simulink model "TST_Rail_CtlLoopLimMeUn"  (R2016b)
settings: Solver=FixedStepDiscrete  StartTime=0.0  StopTime=simTime  FixedStep=sampleTime  RelTol=1e-3
values from neighbouring files (symbols this model uses):
  testCase = 1    [initTST_Rail_CtlLoopLimMeUn_001.m]
libraries: simulink x3, UnitTest_Lib x1
settings Model: Creator=zhengjinyan  LastModifiedBy=zhengjinyan
settings DebuggingCC: SignalRangeChecking=error

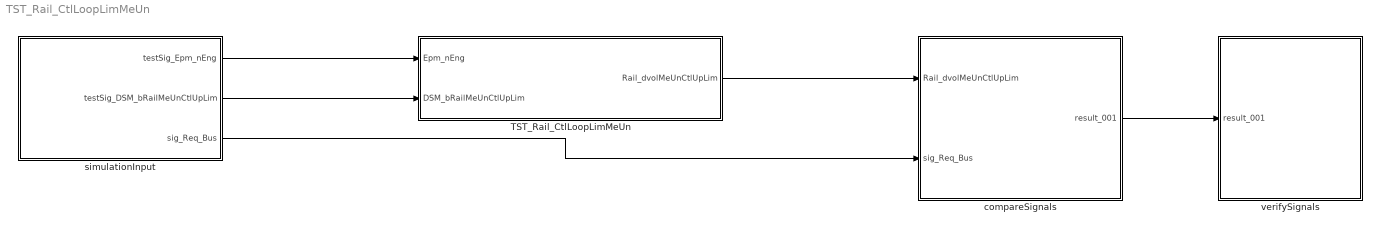
== system TST_Rail_CtlLoopLimMeUn ==
  TST_Rail_CtlLoopLimMeUn : Subsystem
  compareSignals : Subsystem
  simulationInput : Subsystem
  verifySignals : Subsystem
  wires:
  simulationInput/1(testSig_Epm_nEng) -> TST_Rail_CtlLoopLimMeUn/1(Epm_nEng)
  simulationInput/2(testSig_DSM_bRailMeUnCtlUpLim) -> TST_Rail_CtlLoopLimMeUn/2(DSM_bRailMeUnCtlUpLim)
  TST_Rail_CtlLoopLimMeUn/1(Rail_dvolMeUnCtlUpLim) -> compareSignals/1(Rail_dvolMeUnCtlUpLim)
  simulationInput/3(sig_Req_Bus) -> compareSignals/2(sig_Req_Bus)
  compareSignals/1(result_001) -> verifySignals/1(result_001)

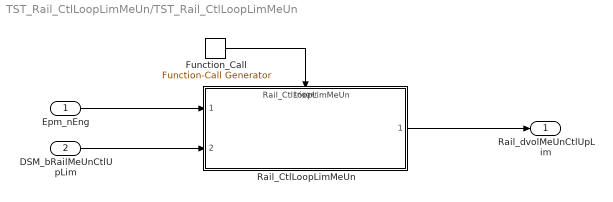
== system TST_Rail_CtlLoopLimMeUn/TST_Rail_CtlLoopLimMeUn ==
  Epm_nEng : Inport
  DSM_bRailMeUnCtlUpLim : Inport  Port=2
  Function_Call : simulink/Ports & Subsystems/Function-Call Generator  sample_time=sampleTime  numberOfIterations=1
  Rail_CtlLoopLimMeUn : ModelReference  ModelNameDialog=Rail_CtlLoopLimMeUn  SimulationMode=Normal  ModelReferenceVersion=1.5  TriggerPortName=function  TriggerPortTriggerType=function-call  TriggerPortStatesWhenEnabling=held
  Rail_dvolMeUnCtlUpLim : Outport
  wires:
  Function_Call/1 -> Rail_CtlLoopLimMeUn/Trigger
  Epm_nEng/1 -> Rail_CtlLoopLimMeUn/1
  DSM_bRailMeUnCtlUpLim/1 -> Rail_CtlLoopLimMeUn/2
  Rail_CtlLoopLimMeUn/1 -> Rail_dvolMeUnCtlUpLim/1

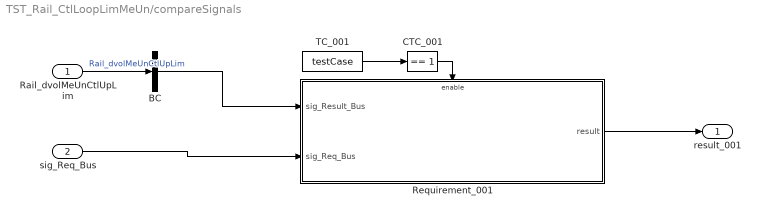
== system TST_Rail_CtlLoopLimMeUn/compareSignals ==
  Rail_dvolMeUnCtlUpLim : Inport
  sig_Req_Bus : Inport  Port=2
  BC : BusCreator  Inputs=1
  CTC_001 : simulink/Logic and Bit Operations/Compare To Constant  relop===  const=1  OutDataTypeStr=boolean
  Requirement_001 : Subsystem
  TC_001 : Constant  Value=testCase
  result_001 : Outport
  wires:
  Rail_dvolMeUnCtlUpLim/1 -> BC/1  "Rail_dvolMeUnCtlUpLim"
  TC_001/1 -> CTC_001/1
  CTC_001/1 -> Requirement_001/Enable
  sig_Req_Bus/1 -> Requirement_001/2(sig_Req_Bus)
  BC/1 -> Requirement_001/1(sig_Result_Bus)
  Requirement_001/1(result) -> result_001/1

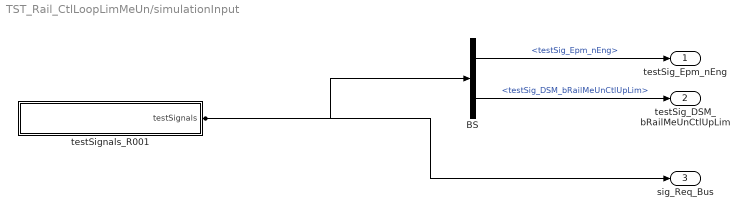
== system TST_Rail_CtlLoopLimMeUn/simulationInput ==
  BS : BusSelector  OutputSignals=testSig_Epm_nEng,testSig_DSM_bRailMeUnCtlUpLim
  testSignals_R001 : Subsystem
  testSig_Epm_nEng : Outport
  testSig_DSM_bRailMeUnCtlUpLim : Outport  Port=2
  sig_Req_Bus : Outport  Port=3
  wires:
  BS/1 -> testSig_Epm_nEng/1  "<testSig_Epm_nEng>"
  BS/2 -> testSig_DSM_bRailMeUnCtlUpLim/1  "<testSig_DSM_bRailMeUnCtlUpLim>"
  testSignals_R001/1(testSignals) -> BS/1, sig_Req_Bus/1

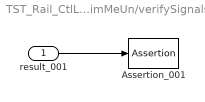
== system TST_Rail_CtlLoopLimMeUn/verifySignals ==
  result_001 : Inport
  Assertion_001 : Assertion  Enabled=off
  wires:
  result_001/1 -> Assertion_001/1

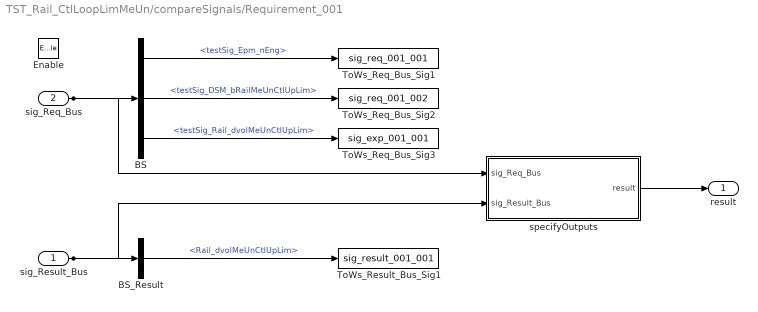
== system TST_Rail_CtlLoopLimMeUn/compareSignals/Requirement_001 ==
  sig_Result_Bus : Inport
  sig_Req_Bus : Inport  Port=2
  Enable : EnablePort
  BS : BusSelector  OutputSignals=testSig_Epm_nEng,testSig_DSM_bRailMeUnCtlUpLim,testSig_Rail_dvolMeUnCtlUpLim
  BS_Result : BusSelector  OutputSignals=Rail_dvolMeUnCtlUpLim
  ToWs_Req_Bus_Sig1 : ToWorkspace  VariableName=sig_req_001_001  SaveFormat=Structure With Time
  ToWs_Req_Bus_Sig2 : ToWorkspace  VariableName=sig_req_001_002  SaveFormat=Structure With Time
  ToWs_Req_Bus_Sig3 : ToWorkspace  VariableName=sig_exp_001_001  SaveFormat=Structure With Time
  ToWs_Result_Bus_Sig1 : ToWorkspace  VariableName=sig_result_001_001  SaveFormat=Structure With Time
  specifyOutputs : Subsystem
  result : Outport
  wires:
  sig_Req_Bus/1 -> BS/1, specifyOutputs/1(sig_Req_Bus)
  BS/1 -> ToWs_Req_Bus_Sig1/1  "<testSig_Epm_nEng>"
  BS/2 -> ToWs_Req_Bus_Sig2/1  "<testSig_DSM_bRailMeUnCtlUpLim>"
  BS/3 -> ToWs_Req_Bus_Sig3/1  "<testSig_Rail_dvolMeUnCtlUpLim>"
  sig_Result_Bus/1 -> BS_Result/1, specifyOutputs/2(sig_Result_Bus)
  BS_Result/1 -> ToWs_Result_Bus_Sig1/1  "<Rail_dvolMeUnCtlUpLim>"
  specifyOutputs/1(result) -> result/1

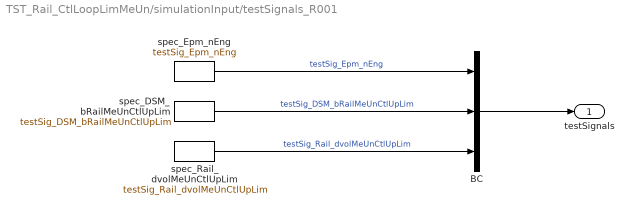
== system TST_Rail_CtlLoopLimMeUn/simulationInput/testSignals_R001 ==
  BC : BusCreator  Inputs=3
  spec_DSM_bRailMeUnCtlUpLim : FromWorkspace  VariableName=testSig_DSM_bRailMeUnCtlUpLim  Interpolate=off  OutputAfterFinalValue=Holding final value
  spec_Epm_nEng : FromWorkspace  VariableName=testSig_Epm_nEng  Interpolate=off  OutputAfterFinalValue=Holding final value
  spec_Rail_dvolMeUnCtlUpLim : FromWorkspace  VariableName=testSig_Rail_dvolMeUnCtlUpLim  Interpolate=off  OutputAfterFinalValue=Holding final value
  testSignals : Outport
  wires:
  BC/1 -> testSignals/1
  spec_Epm_nEng/1 -> BC/1  "testSig_Epm_nEng"
  spec_DSM_bRailMeUnCtlUpLim/1 -> BC/2  "testSig_DSM_bRailMeUnCtlUpLim"
  spec_Rail_dvolMeUnCtlUpLim/1 -> BC/3  "testSig_Rail_dvolMeUnCtlUpLim"

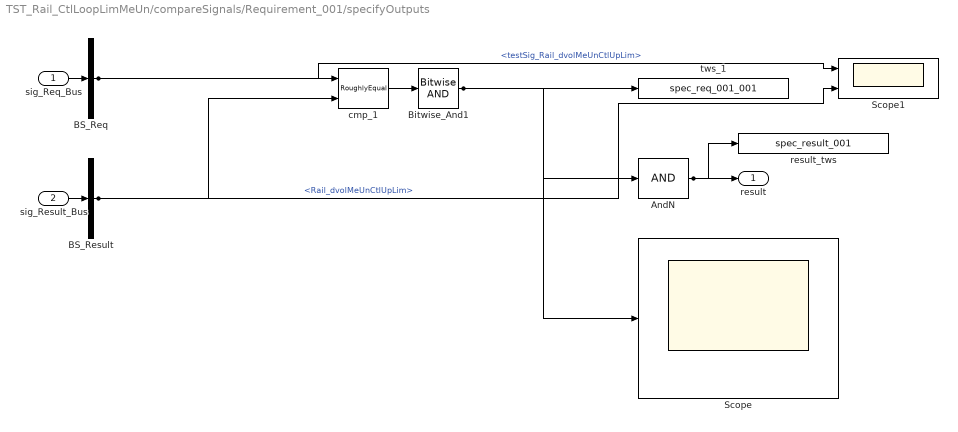
== system TST_Rail_CtlLoopLimMeUn/compareSignals/Requirement_001/specifyOutputs ==
  sig_Req_Bus : Inport
  sig_Result_Bus : Inport  Port=2
  AndN : Logic  Inputs=1
  BS_Req : BusSelector  OutputSignals=testSig_Rail_dvolMeUnCtlUpLim
  BS_Result : BusSelector  OutputSignals=Rail_dvolMeUnCtlUpLim
  Bitwise_And1 : simulink/Logic and Bit Operations/Bitwise Operator  logicop=AND  UseBitMask=off  BitMask=bin2dec('11011001')  BitMaskRealWorld=Stored Integer
  Scope : Scope
  Scope1 : Scope  NumInputPorts=2
  cmp_1 : UnitTest_Lib/RoughlyEqual  slope=0.1
  result_tws : ToWorkspace  VariableName=spec_result_001
  tws_1 : ToWorkspace  VariableName=spec_req_001_001
  result : Outport
  wires:
  sig_Req_Bus/1 -> BS_Req/1
  sig_Result_Bus/1 -> BS_Result/1
  AndN/1 -> result/1, result_tws/1
  BS_Req/1 -> cmp_1/1, Scope1/1  "<testSig_Rail_dvolMeUnCtlUpLim>"
  BS_Result/1 -> cmp_1/2, Scope1/2  "<Rail_dvolMeUnCtlUpLim>"
  cmp_1/1 -> Bitwise_And1/1
  Bitwise_And1/1 -> tws_1/1, AndN/1, Scope/1
